simulink model "classic"  (R2020b)
settings: Solver=VariableStepAuto  StartTime=0.0  StopTime=10.0  RelTol=1e-3
settings Model: Creator=mluser  LastModifiedBy=mluser

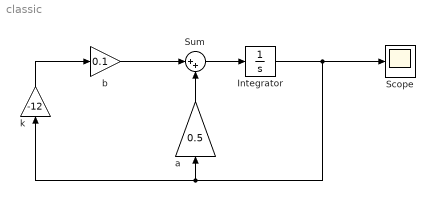
== system classic ==
  Integrator : Integrator  InitialCondition=1
  Scope : Scope
  Sum : Sum  Inputs=|++
  a : Gain  Gain=0.5
  b : Gain  Gain=0.1
  k : Gain  Gain=-12
  wires:
  k/1 -> b/1
  b/1 -> Sum/1
  a/1 -> Sum/2
  Sum/1 -> Integrator/1
  Integrator/1 -> k/1, a/1, Scope/1
